simulink model "Bicopter_Dynamics"  (R2019a)
settings: Solver=ode4  StartTime=0.0  StopTime=5  FixedStep=0.00001  RelTol=1e-3
settings Model: Creator=crsmyth  LastModifiedBy=crs20

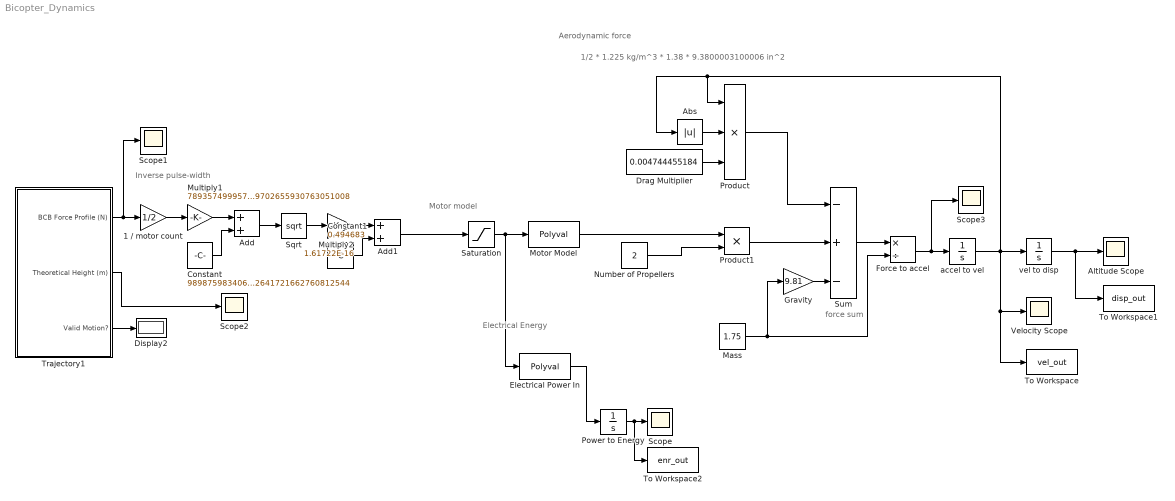
== system Bicopter_Dynamics ==
  note: Inverse pulse-width
  note: Electrical Energy
  note: force sum
  note: Motor model
  note: Aerodynamic force
  note: 1/2 * 1.225 kg/m^3 * 1.38 * 9.3800003100006 in^2
  1 / motor count : Gain  Gain=1/2
  Abs : Abs
  Add : Sum
  Add1 : Sum
  Altitude Scope : Scope
  Constant : Constant  Value=9898759834062641721662760812544
  Constant1 : Constant  Value=0.494683
  Display2 : Display
  Drag Multiplier : Constant  Value=0.004744455184
  Electrical Power In : Polyval  Coefs=[2.956191832898671e+02, -6.235353126465623e+02, 3.330393150826374e+02]
  Force to accel : Product  Inputs=*/
  Gravity : Gain  Gain=9.81
  Mass : Constant  Value=1.75
  Motor Model : Polyval  Coefs=[4.843819998761814,-4.792311105872948,-0.068689974553541]
  Multiply1 : Gain  Gain=7893574999579702655930763051008
  Multiply2 : Gain  Gain=1.61722E-16
  Number of Propellers : Constant  Value=2
  Power to Energy : Integrator
  Product : Product  Inputs=3
  Product1 : Product
  Saturation : Saturate  UpperLimit=2  LowerLimit=1
  Scope{,1..3} (4 alike) : Scope
  Sqrt : Sqrt  SaturateOnIntegerOverflow=on
  Sum : Sum  Inputs=-+-
  To Workspace : ToWorkspace  VariableName=vel_out  SampleTime=-1
      settings: Save2DSignal=2-D array (concatenate along first dimension)
  To Workspace1 : ToWorkspace  VariableName=disp_out  SampleTime=-1
      settings: Save2DSignal=2-D array (concatenate along first dimension)
  To Workspace2 : ToWorkspace  VariableName=enr_out  SaveFormat=Timeseries  SampleTime=-1
  Trajectory1 : Subsystem  mask{fA=1, dT=4, xF=2, mass=1.75}
      mask prompts: fA "Max Force Pulse Amplitude (N)"; dT "Desired Maneuver time (sec)"; xF "Height Change (m)"; mass "Mass of Copter (kg)"
  Velocity Scope : Scope
  accel to vel : Integrator
  vel to disp : Integrator
  wires:
  Sum/1 -> Force to accel/1
  Mass/1 -> Gravity/1, Force to accel/2
  Gravity/1 -> Sum/3
  Product/1 -> Sum/1
  Drag Multiplier/1 -> Product/3
  Abs/1 -> Product/2
  Product1/1 -> Sum/2
  Number of Propellers/1 -> Product1/2
  Motor Model/1 -> Product1/1
  accel to vel/1 -> vel to disp/1, Abs/1, Product/1, To Workspace/1, Velocity Scope/1
  vel to disp/1 -> To Workspace1/1, Altitude Scope/1
  Electrical Power In/1 -> Power to Energy/1
  Power to Energy/1 -> To Workspace2/1, Scope/1
  Saturation/1 -> Electrical Power In/1, Motor Model/1
  Add1/1 -> Saturation/1
  Trajectory1/3(Valid Motion?) -> Display2/1
  Trajectory1/1(BCB Force Profile (N)) -> Scope1/1, 1 / motor count/1
  1 / motor count/1 -> Multiply1/1
  Multiply1/1 -> Add/1
  Constant/1 -> Add/2
  Add/1 -> Sqrt/1
  Sqrt/1 -> Multiply2/1
  Multiply2/1 -> Add1/1
  Constant1/1 -> Add1/2
  Trajectory1/2(Theoretical Height (m)) -> Scope2/1
  Force to accel/1 -> Scope3/1, accel to vel/1

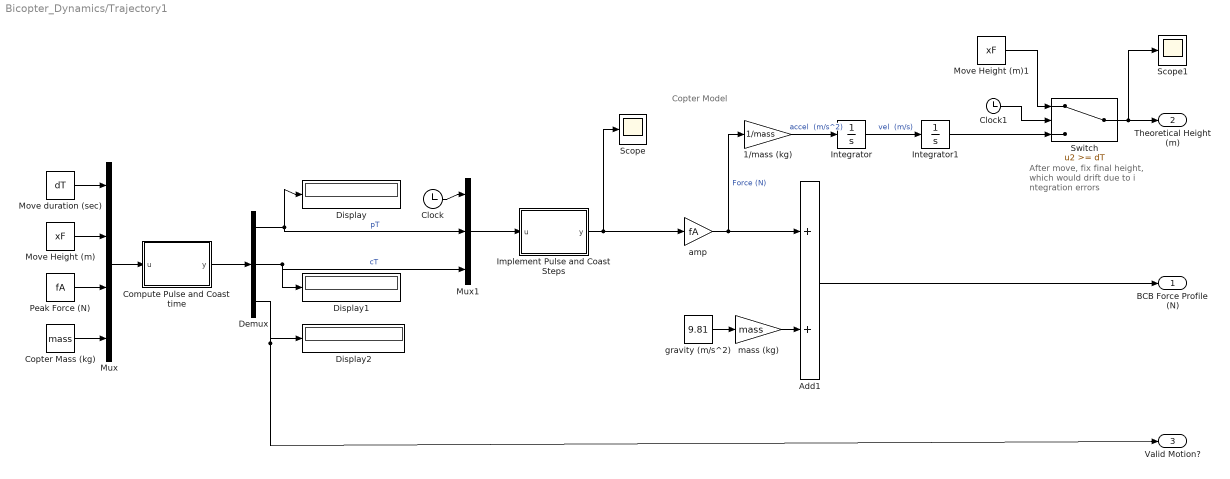
== system Bicopter_Dynamics/Trajectory1 ==
  note: After move, fix final height,
      | which would drift due to i
      | ntegration errors
  note: Copter Model
  1/mass (kg) : Gain  Gain=1/mass
  Add1 : Sum
  Clock : Clock
  Clock1 : Clock
  Compute Pulse and Coast time : MATLAB Function  TreatAsAtomicUnit=on
  Copter Mass (kg) : Constant  Value=mass
  Demux : Demux  Outputs=3
  Display : Display
  Display1 : Display
  Display2 : Display
  Implement Pulse and Coast Steps : MATLAB Function  TreatAsAtomicUnit=on
  Integrator : Integrator
  Integrator1 : Integrator
  Move Height (m)1 : Constant  Value=xF
  Move Height (m) : Constant  Value=xF
  Move duration (sec) : Constant  Value=dT
  Mux : Mux
  Mux1 : Mux  Inputs=3
  "Peak Force (N) " : Constant  Value=fA
  Scope : Scope
  Scope1 : Scope
  Switch : Switch  Threshold=dT
  amp : Gain  Gain=fA
  gravity (m/s^2) : Constant  Value=9.81
  mass (kg) : Gain  Gain=mass
  BCB Force Profile (N) : Outport
  Theoretical Height (m) : Outport  Port=2
  Valid Motion? : Outport  Port=3
  wires:
  Add1/1 -> BCB Force Profile (N)/1
  Compute Pulse and Coast time/1(y) -> Demux/1
  Demux/1 -> Display/1, Mux1/2  "pT"
  Demux/2 -> Display1/1, Mux1/3  "cT"
  Move duration (sec)/1 -> Mux/1
  Move Height (m)/1 -> Mux/2
  "Peak Force (N) "/1 -> Mux/3
  Copter Mass (kg)/1 -> Mux/4
  Mux/1 -> Compute Pulse and Coast time/1(u)
  amp/1 -> Add1/1, 1/mass (kg)/1  "Force (N)"
  gravity (m/s^2)/1 -> mass (kg)/1
  1/mass (kg)/1 -> Integrator/1  "accel  (m/s^2)"
  mass (kg)/1 -> Add1/2
  Switch/1 -> Theoretical Height (m)/1, Scope1/1
  Integrator/1 -> Integrator1/1  "vel  (m/s)"
  Clock/1 -> Mux1/1
  Mux1/1 -> Implement Pulse and Coast Steps/1(u)
  Implement Pulse and Coast Steps/1(y) -> Scope/1, amp/1
  Demux/3 -> Valid Motion?/1, Display2/1
  Clock1/1 -> Switch/2
  Integrator1/1 -> Switch/3
  Move Height (m)1/1 -> Switch/1

== matlab function Bicopter_Dynamics/Trajectory1/Implement Pulse and Coast Steps ==
  data: u input; y output
function y = fcn(u)
%#codegen


t  = u(1);
pT = u(2);
cT = u(3);

if(t >= pT)
  a = -1;
else
  a = 0;
end

if(t >= pT+cT)
  b = -1;
else
  b = 0;
end

if(t >= 2*pT+cT)
  c = 1;
else
  c = 0;
end

y = 1 + a + b + c;

== matlab function Bicopter_Dynamics/Trajectory1/Compute Pulse and Coast time ==
  data: u input; y output
function y = fcn(u)
%#codegen

% Gordon Parker
% Michigan Technological University
% 08 Jan 2015

% Modified by Eddy Trinklein
% 27 Sept 2016


% calculates a bang-coast-bang force input to move the copter from
% rest to rest vertically. 
%
% Dialog inputs:
% dT:   desired maneuver time (sec)
% xF:   altitude change (m)
% fA:   desired force amplitude (N)
% mass: mass of copter (kg)

% Outputs:
% pTActual:  Computed pulse times (sec)
% cTActual:  coast time (sec)


dT   = u(1);
xF   = u(2);
fA   = u(3);
mass = u(4);

y = zeros(1,3);

aA = fA/mass;


tmp1 = dT^2 - 4*xF/aA;
if tmp1 < 0
  dTWorks = sqrt(4*xF/aA);
  aAWorks = 4*xF/dT^2;
  xFWorks = fA/4*dT^2;
  fprintf('This set of inputs will not work you can either:\n');
  fprintf('1) Use a maneuver time of %f\n',dTWorks);
  fprintf('2) Use a force amplitude of %f\n',aAWorks*mass);
  fprintf('3) Use a final distance of %f\n',xFWorks);
  y = [.1,.1,0];
  return;
end

%% Create Solution

% Calc pulse times that work
pT = roots([1 -dT xF/aA]); % (sec)

% pick the shortest duration pulse
pTActual = min(pT); % (sec)

% set coast time
cTActual = dT - 2*pTActual; % (sec)
  

y = [real(pTActual),real(cTActual),1];
